simulink model "Modelo_estados_practica7"  (R2021a)
settings: Solver=FixedStepAuto  StartTime=0.0  StopTime=5  FixedStep=0.001  RelTol=1e-3
libraries: cstblocks x1, simulink x1
settings Model: Creator=faust  LastModifiedBy=joaqu

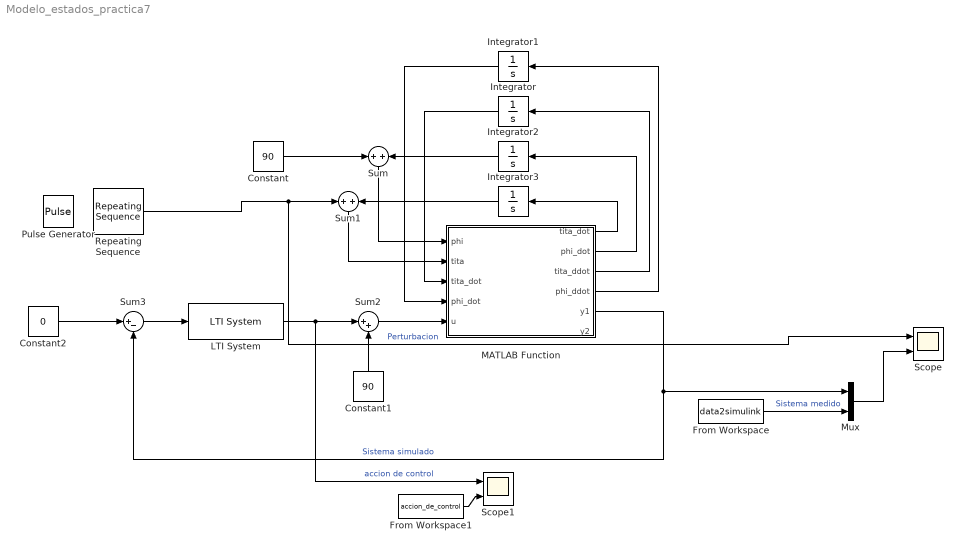
== system Modelo_estados_practica7 ==
  Constant : Constant  Value=90
  Constant1 : Constant  Value=90
  Constant2 : Constant  Value=0
  From Workspace : FromWorkspace  VariableName=data2simulink  SampleTime=0.01
  From Workspace1 : FromWorkspace  VariableName=accion_de_control  SampleTime=0.01
  Integrator{,1..3} (4 alike) : Integrator
  LTI System : cstblocks/LTI System  sys=Cd_p  IC=[]
  MATLAB Function : MATLAB Function  TreatAsAtomicUnit=on
  Mux : Mux  Inputs=2
  Pulse Generator : DiscretePulseGenerator  PulseType=Time based  Amplitude=30  Period=5  PhaseDelay=0.079
  Repeating Sequence : simulink/Sources/Repeating Sequence  rep_seq_t=[0 0.08 0.24 0.25 0.36 5]  rep_seq_y=[0 0 30 30 0 0]
  Scope : Scope  NumInputPorts=2
  Scope1 : Scope  NumInputPorts=2
  Sum : Sum  Inputs=+|+
  Sum1 : Sum  Inputs=+|+
  Sum2 : Sum  Inputs=|++
  Sum3 : Sum  Inputs=|+-
  wires:
  MATLAB Function/3(tita_ddot) -> Integrator/1
  Integrator/1 -> MATLAB Function/3("tita_dot ")
  MATLAB Function/5(y1) -> Mux/1, Sum3/2  "Sistema simulado"
  MATLAB Function/4(phi_ddot) -> Integrator1/1
  Integrator1/1 -> MATLAB Function/4("phi_dot ")
  MATLAB Function/1(tita_dot) -> Integrator3/1
  MATLAB Function/2(phi_dot) -> Integrator2/1
  Sum1/1 -> MATLAB Function/2(tita)
  Integrator3/1 -> Sum1/2
  Constant/1 -> Sum/1
  Sum/1 -> MATLAB Function/1(phi)
  Integrator2/1 -> Sum/2
  Constant2/1 -> Sum3/1
  LTI System/1 -> Scope1/1, Sum2/1  "accion de control"
  Sum2/1 -> MATLAB Function/5(u)
  Constant1/1 -> Sum2/2
  Sum3/1 -> LTI System/1
  From Workspace/1 -> Mux/2  "Sistema medido"
  Mux/1 -> Scope/2
  Repeating Sequence/1 -> Scope/1, Sum1/1  "Perturbacion"
  From Workspace1/1 -> Scope1/2

== matlab function Modelo_estados_practica7/MATLAB Function ==
  data: tita_dot output; phi_dot output; phi input; tita input; tita_dot input; phi_dot input; tita_ddot output; phi_ddot output; u input; y1 output; y2 output
function [tita_dot,phi_dot,tita_ddot,phi_ddot,y1, y2] = fcn(phi, tita, tita_dot,phi_dot,u)

a = 0.7;
b = 2.613;
c = 65;
d = 292.2;
e = 30.67;
f = d;

phi_ddot = d * u - e * phi_dot - f * phi;
tita_ddot = phi_ddot * a - b * tita_dot - c * tita;

y1 = tita;
y2 = phi;
